simulink model "diagrama_completo"  (R2020b)
settings: Solver=VariableStepAuto  StartTime=0.0  StopTime=25  MaxStep=1e-4  RelTol=1e-4
model workspace (MAT data in the model file):
  Cts = 0.818
  Jeq = 5.65099476805e-06
  Ld = 0.0066
  Lls = 0.0008
  Lq = 0.0058
  Pp = 3
  Rs = 1.02
  Rts_amb = 146.7
  beq = 1.5e-05
  lambda_m = 0.01546
  r = 314.3008
  ws = 15000
  wsv = 30000
values from neighbouring files (symbols this model uses):
  ba = Jeq*n*wpos    (= 0.0113019895361)    [valores.m]
  kotheta = 3*pobs    (= 9600)    [valores.m]
  koTl = (pobs^3)    (= 32768000000)    [valores.m]
  kow = 3*(pobs^2)    (= 30720000)    [valores.m]
  ksa = ba*wpos    (= 9.04159162887)    [valores.m]
  ksia = ksa*wint    (= 2893.30932124)    [valores.m]
  R0 = Lls*pi    (= 4)    [valores.m]
  Rd = Ld*pi    (= 33)    [valores.m]
  Rq = Lq*pi    (= 29)    [valores.m]
undefined symbols (not defined in the file or in its folder): sigbuilder_block
(part 2 of 2)

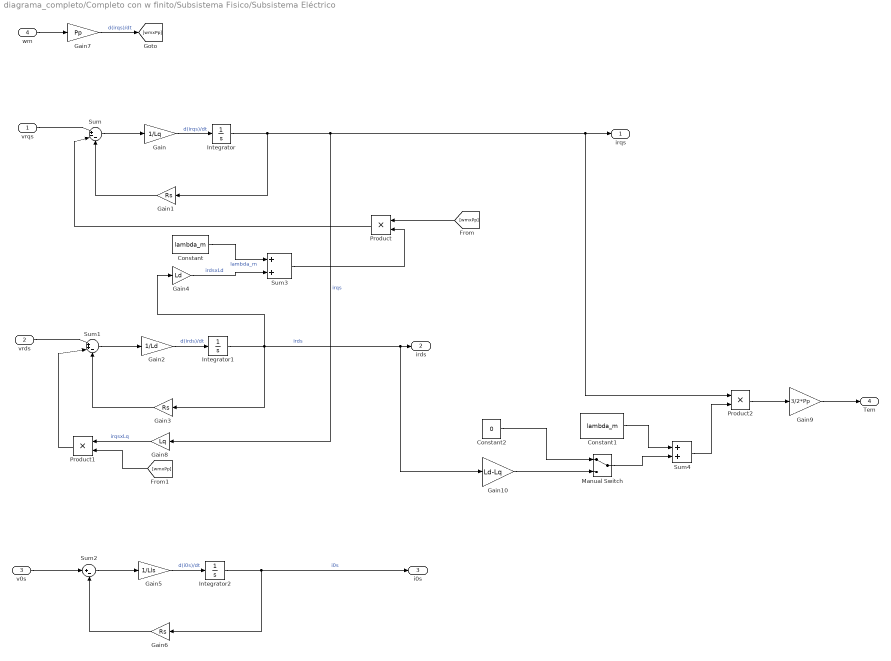
== system diagrama_completo/Completo con w finito/Subsistema Fisico/Subsistema Eléctrico ==
  vrqs : Inport
  vrds : Inport  Port=2
  v0s : Inport  Port=3
  wm : Inport  Port=4
  Constant : Constant  Value=lambda_m
  Constant1 : Constant  Value=lambda_m
  Constant2 : Constant  Value=0
  Gain : Gain  Gain=1/Lq
  Gain1 : Gain  Gain=Rs
  Gain10 : Gain  Gain=Ld-Lq
  Gain2 : Gain  Gain=1/Ld
  Gain3 : Gain  Gain=Rs
  Gain4 : Gain  Gain=Ld
  Gain5 : Gain  Gain=1/Lls
  Gain6 : Gain  Gain=Rs
  Gain7 : Gain  Gain=Pp
  Gain8 : Gain  Gain=Lq
  Gain9 : Gain  Gain=3/2*Pp
  Integrator : Integrator
  Integrator1 : Integrator
  Integrator2 : Integrator
  Manual Switch : ManualSwitch
  Product : Product
  Product1 : Product
  Product2 : Product
  Sum : Sum  Inputs=|+--
  Sum1 : Sum  Inputs=|++-
  Sum2 : Sum  Inputs=|+-
  Sum3 : Sum
  Sum4 : Sum
  irqs : Outport
  irds : Outport  Port=2
  i0s : Outport  Port=3
  Tem : Outport  Port=4
  wires:
  Integrator1/1 -> Gain4/1, Gain3/1, Gain10/1, irds/1  "irds"
  Gain2/1 -> Integrator1/1  "d(irds)/dt"
  Gain3/1 -> Sum1/3
  vrqs/1 -> Sum/1
  vrds/1 -> Sum1/1
  v0s/1 -> Sum2/1
  Gain5/1 -> Integrator2/1  "d(i0s)/dt"
  Integrator2/1 -> Gain6/1, i0s/1  "i0s"
  Gain1/1 -> Sum/3
  Integrator/1 -> Gain1/1, Gain8/1, Product2/1, irqs/1  "irqs"
  Gain/1 -> Integrator/1  "d(irqs)/dt"
  Gain6/1 -> Sum2/2
  Gain4/1 -> Sum3/2  "irdsxLd"
  Constant/1 -> Sum3/1  "lambda_m"
  wm/1 -> Gain7/1
  Gain7/1 -> [wmxPp]  "d(irqs)/dt"
  [wmxPp] -> Product/1
  Product/1 -> Sum/2
  Sum3/1 -> Product/2
  Gain8/1 -> Product1/1  "irqsxLq"
  [wmxPp] -> Product1/2
  Product1/1 -> Sum1/2
  Constant1/1 -> Sum4/1
  Sum4/1 -> Product2/2
  Product2/1 -> Gain9/1
  Gain9/1 -> Tem/1
  Sum/1 -> Gain/1
  Sum1/1 -> Gain2/1
  Sum2/1 -> Gain5/1
  Gain10/1 -> Manual Switch/2
  Constant2/1 -> Manual Switch/1
  Manual Switch/1 -> Sum4/2

== system diagrama_completo/Completo con w finito/Subsistema Fisico/Subsistema Mecánico ==
  Tl : Inport
  Tem : Inport  Port=2
  Gain : Gain  Gain=1/Jeq
  Gain1 : Gain  Gain=beq
  Gain2 : Gain  Gain=1/r
  Integrator : Integrator
  Integrator1 : Integrator
  Sum : Sum  Inputs=-+-
  wm : Outport
  theta_m : Outport  Port=2
  wires:
  Sum/1 -> Gain/1
  Tl/1 -> Gain2/1
  Gain1/1 -> Sum/3
  Integrator/1 -> Gain1/1, wm/1, Integrator1/1  "wm"
  Gain2/1 -> Sum/1
  Gain/1 -> Integrator/1  "acel"
  Integrator1/1 -> theta_m/1  "theta_m"
  Tem/1 -> Sum/2

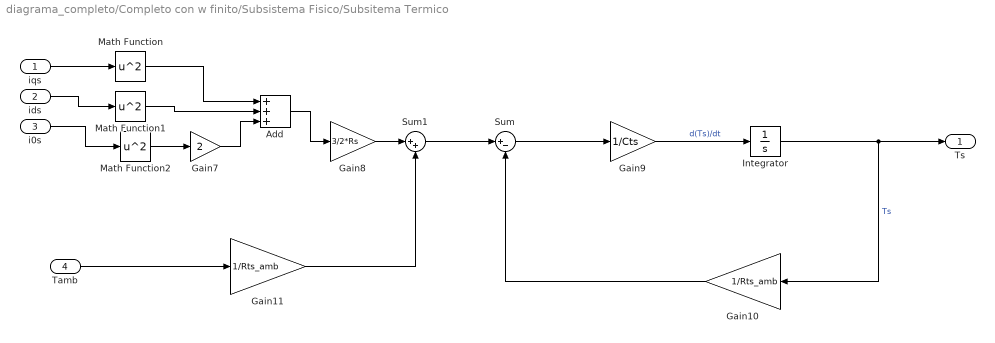
== system diagrama_completo/Completo con w finito/Subsistema Fisico/Subsitema Termico ==
  iqs : Inport
  ids : Inport  Port=2
  i0s : Inport  Port=3
  Tamb : Inport  Port=4
  Add : Sum  Inputs=+++
  Gain10 : Gain  Gain=1/Rts_amb
  Gain11 : Gain  Gain=1/Rts_amb
  Gain7 : Gain  Gain=2
  Gain8 : Gain  Gain=3/2*Rs
  Gain9 : Gain  Gain=1/Cts
  Integrator : Integrator  InitialCondition=40
  Math Function : Math  Operator=square  SaturateOnIntegerOverflow=on
  Math Function1 : Math  Operator=square  SaturateOnIntegerOverflow=on
  Math Function2 : Math  Operator=square  SaturateOnIntegerOverflow=on
  Sum : Sum  Inputs=|+-
  Sum1 : Sum  Inputs=|++
  Ts : Outport
  wires:
  Gain11/1 -> Sum1/2
  Gain8/1 -> Sum1/1
  Add/1 -> Gain8/1
  Gain9/1 -> Integrator/1  "d(Ts)/dt"
  Gain10/1 -> Sum/2
  Integrator/1 -> Gain10/1, Ts/1  "Ts"
  i0s/1 -> Math Function2/1
  Math Function/1 -> Add/1
  ids/1 -> Math Function1/1
  Sum1/1 -> Sum/1
  Gain7/1 -> Add/3
  Sum/1 -> Gain9/1
  Tamb/1 -> Gain11/1
  Math Function2/1 -> Gain7/1
  iqs/1 -> Math Function/1
  Math Function1/1 -> Add/2

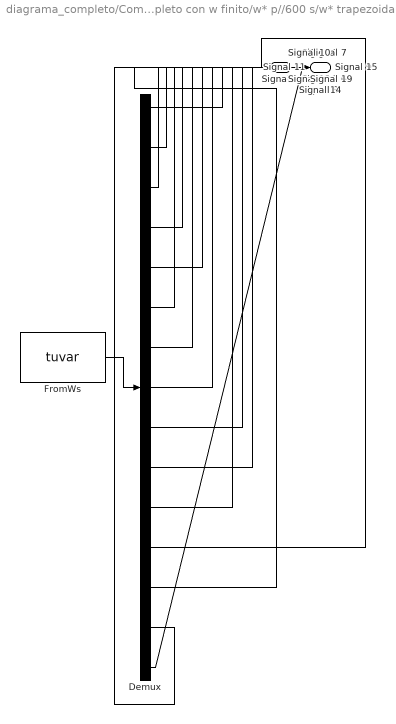
== system diagrama_completo/Completo con w finito/w* p//600 s/w* trapezoidal1 ==
  Demux : Demux  Tag=STV Demux  Outputs=15
      settings: DisplayOption=none
  FromWs : FromWorkspace  Tag=STV FromWs  VariableName=tuvar
      SigBuilderData=|
      | common.afterFinalStr = 'Extrapolate'
      | common.sampleTime = 0
      | dataSet.timeRange = [0 155]
      | dataSet.name = 'Group 1'
      | sbobj.Groups.Name = 'Group 1'
      | sbobj.Groups.Signals(1).Name = 'Signal 1'
      | sbobj.Groups.Signals(1).XData = [0 5 5.2 9.8 10 155]
      | sbobj.Groups.Signals(1).YData = [0 0 1.25663706144 1.25663706144 0 0]
      | sbobj.Groups.Signals(2).Name = 'Signal 2'
      | sbobj.Groups.Signals(2).XData = [0 15 15.2 19.8 20 155]
      | sbobj.Groups.Signals(2).YData = [0 0 -1.25663706144 -1.25663706144 0 0]
      | sbobj.Groups.Signals(3).Name = 'Signal 3'
      | sbobj.Groups.Signals(3).XData = [0 25 25.2 29.8 30 155]
      | sbobj.Groups.Signals(3).YData = [0 0 1.25663706144 1.25663706144 0 0]
      | sbobj.Groups.Signals(4).Name = 'Signal 4'
      | sbobj.Groups.Signals(4).XData = [0 35 35.2 39.8 40 155]
      | sbobj.Groups.Signals(4).YData = [0 0 -1.25663706144 -1.25663706144 0 0]
      | sbobj.Groups.Signals(5).Name = 'Signal 5'
      | sbobj.Groups.Signals(5).XData = [0 45 45.2 49.8 50 155]
      | sbobj.Groups.Signals(5).YData = [0 0 1.25663706144 1.25663706144 0 0]
      | sbobj.Groups.Signals(6).Name = 'Signal 6'
      | sbobj.Groups.Signals(6).XData = [0 55 55.2 59.8 60 155]
      | sbobj.Groups.Signals(6).YData = [0 0 -1.25663706144 -1.25663706144 0 0]
      | sbobj.Groups.Signals(7).Name = 'Signal 7'
      | sbobj.Groups.Signals(7).XData = [0 65 65.2 69.8 70 155]
      | sbobj.Groups.Signals(7).YData = [0 0 1.25663706144 1.25663706144 0 0]
      | sbobj.Groups.Signals(8).Name = 'Signal 8'
      | sbobj.Groups.Signals(8).XData = [0 75 75.2 79.8 80 155]
      | sbobj.Groups.Signals(8).YData = [0 0 -1.25663706144 -1.25663706144 0 0]
      | sbobj.Groups.Signals(9).Name = 'Signal 9'
      | sbobj.Groups.Signals(9).XData = [0 85 85.2 89.8 90 155]
      | sbobj.Groups.Signals(9).YData = [0 0 1.25663706144 1.25663706144 0 0]
      | sbobj.Groups.Signals(10).Name = 'Signal 10'
      | sbobj.Groups.Signals(10).XData = [0 95 95.2 99.8 100 155]
      | sbobj.Groups.Signals(10).YData = [0 0 -1.25663706144 -1.25663706144 0 0]
      | sbobj.Groups.Signals(11).Name = 'Signal 11'
      | sbobj.Groups.Signals(11).XData = [0 105 105.2 109.8 110 155]
      | sbobj.Groups.Signals(11).YData = [0 0 1.25663706144 1.25663706144 0 0]
      | sbobj.Groups.Signals(12).Name = 'Signal 12'
      | sbobj.Groups.Signals(12).XData = [0 115 115.2 119.8 120 155]
      | sbobj.Groups.Signals(12).YData = [0 0 -1.25663706144 -1.25663706144 0 0]
      | sbobj.Groups.Signals(13).Name = 'Signal 14'
      | sbobj.Groups.Signals(13).XData = [0 125 125.2 129.8 130 155]
      | sbobj.Groups.Signals(13).YData = [0 0 1.2566 1.2566 0 0]
      | sbobj.Groups.Signals(14).Name = 'Signal 15'
      | sbobj.Groups.Signals(14).XData = [0 135 135.2 139.8 140 155]
      | sbobj.Groups.Signals(14).YData = [0 0 -1.2566 -1.2566 0 0]
      | sbobj.Groups.Signals(15).Name = 'Signal 19'
      | sbobj.Groups.Signals(15).XData = [0 145 145.2 149.8 150 155]
      | sbobj.Groups.Signals(15).YData = [0 0 1.2566 1.2566 0 0]
      | sbobj.Groups.TimeRange = [0 155]
  Signal 1 : Outport  Tag=STV Outport
  Signal 2 : Outport  Tag=STV Outport  Port=2
  Signal 3 : Outport  Tag=STV Outport  Port=3
  Signal 4 : Outport  Tag=STV Outport  Port=4
  Signal 5 : Outport  Tag=STV Outport  Port=5
  Signal 6 : Outport  Tag=STV Outport  Port=6
  Signal 7 : Outport  Tag=STV Outport  Port=7
  Signal 8 : Outport  Tag=STV Outport  Port=8
  Signal 9 : Outport  Tag=STV Outport  Port=9
  Signal 10 : Outport  Tag=STV Outport  Port=10
  Signal 11 : Outport  Tag=STV Outport  Port=11
  Signal 12 : Outport  Tag=STV Outport  Port=12
  Signal 14 : Outport  Tag=STV Outport  Port=13
  Signal 15 : Outport  Tag=STV Outport  Port=14
  Signal 19 : Outport  Tag=STV Outport  Port=15
  wires:
  FromWs/1 -> Demux/1
  Demux/1 -> Signal 1/1
  Demux/2 -> Signal 2/1
  Demux/3 -> Signal 3/1
  Demux/4 -> Signal 4/1
  Demux/5 -> Signal 5/1
  Demux/6 -> Signal 6/1
  Demux/7 -> Signal 7/1
  Demux/8 -> Signal 8/1
  Demux/9 -> Signal 9/1
  Demux/10 -> Signal 10/1
  Demux/11 -> Signal 11/1
  Demux/12 -> Signal 12/1
  Demux/13 -> Signal 14/1
  Demux/14 -> Signal 15/1
  Demux/15 -> Signal 19/1

== system diagrama_completo/Completo con w finito/w* p//600 s/w* trapezoidal2 ==
  Demux : Demux  Tag=STV Demux  Outputs=15
      settings: DisplayOption=none
  FromWs : FromWorkspace  Tag=STV FromWs  VariableName=tuvar
      SigBuilderData=|
      | common.afterFinalStr = 'Extrapolate'
      | common.sampleTime = 0
      | dataSet.timeRange = [0 305]
      | dataSet.name = 'Group 1'
      | sbobj.Groups.Name = 'Group 1'
      | sbobj.Groups.Signals(1).Name = 'Signal 1'
      | sbobj.Groups.Signals(1).XData = [0 155 155.2 159.8 160 305]
      | sbobj.Groups.Signals(1).YData = [0 0 -1.2566 -1.25663706144 0 0]
      | sbobj.Groups.Signals(2).Name = 'Signal 2'
      | sbobj.Groups.Signals(2).XData = [0 165 165.2 169.8 170 305]
      | sbobj.Groups.Signals(2).YData = [0 0 1.2566 1.2566 0 0]
      | sbobj.Groups.Signals(3).Name = 'Signal 3'
      | sbobj.Groups.Signals(3).XData = [0 175 175.2 179.8 180 305]
      | sbobj.Groups.Signals(3).YData = [0 0 -1.25663706144 -1.2566 0 0]
      | sbobj.Groups.Signals(4).Name = 'Signal 4'
      | sbobj.Groups.Signals(4).XData = [0 185 185.2 189.8 190 305]
      | sbobj.Groups.Signals(4).YData = [0 0 1.2566 1.2566 0 0]
      | sbobj.Groups.Signals(5).Name = 'Signal 5'
      | sbobj.Groups.Signals(5).XData = [0 195 195.2 199.8 200 305]
      | sbobj.Groups.Signals(5).YData = [0 0 -1.2566 -1.2566 0 0]
      | sbobj.Groups.Signals(6).Name = 'Signal 6'
      | sbobj.Groups.Signals(6).XData = [0 205 205.2 209.8 210 305]
      | sbobj.Groups.Signals(6).YData = [0 0 1.2566 1.2566 0 0]
      | sbobj.Groups.Signals(7).Name = 'Signal 7'
      | sbobj.Groups.Signals(7).XData = [0 215 215.2 219.8 220 305]
      | sbobj.Groups.Signals(7).YData = [0 0 -1.2566 -1.2566 0 0]
      | sbobj.Groups.Signals(8).Name = 'Signal 8'
      | sbobj.Groups.Signals(8).XData = [0 225 225.2 229.8 230 305]
      | sbobj.Groups.Signals(8).YData = [0 0 1.2566 1.2566 0 0]
      | sbobj.Groups.Signals(9).Name = 'Signal 9'
      | sbobj.Groups.Signals(9).XData = [0 235 235.2 239.8 240 305]
      | sbobj.Groups.Signals(9).YData = [0 0 -1.2566 -1.2566 0 0]
      | sbobj.Groups.Signals(10).Name = 'Signal 10'
      | sbobj.Groups.Signals(10).XData = [0 245 245.2 249.8 250 305]
      | sbobj.Groups.Signals(10).YData = [0 0 1.25663706144 1.2566 0 0]
      | sbobj.Groups.Signals(11).Name = 'Signal 11'
      | sbobj.Groups.Signals(11).XData = [0 255 255.2 259.8 260 305]
      | sbobj.Groups.Signals(11).YData = [0 0 -1.2566 -1.2566 0 0]
      | sbobj.Groups.Signals(12).Name = 'Signal 12'
      | sbobj.Groups.Signals(12).XData = [0 265 265.2 269.8 270 305]
      | sbobj.Groups.Signals(12).YData = [0 0 1.2566 1.2566 0 0]
      | sbobj.Groups.Signals(13).Name = 'Signal 13'
      | sbobj.Groups.Signals(13).XData = [0 275 275.2 279.8 280 305]
      | sbobj.Groups.Signals(13).YData = [0 0 -1.2566 -1.2566 0 0]
      | sbobj.Groups.Signals(14).Name = 'Signal 14'
      | sbobj.Groups.Signals(14).XData = [0 285 285.2 289.8 290 305]
      | sbobj.Groups.Signals(14).YData = [0 0 1.2566 1.2566 0 0]
      | sbobj.Groups.Signals(15).Name = 'Signal 15'
      | sbobj.Groups.Signals(15).XData = [0 295 295.2 299.8 300 305]
      | sbobj.Groups.Signals(15).YData = [0 0 -1.2566 -1.2566 0 0]
      | sbobj.Groups.TimeRange = [0 305]
  Signal 1 : Outport  Tag=STV Outport
  Signal 2 : Outport  Tag=STV Outport  Port=2
  Signal 3 : Outport  Tag=STV Outport  Port=3
  Signal 4 : Outport  Tag=STV Outport  Port=4
  Signal 5 : Outport  Tag=STV Outport  Port=5
  Signal 6 : Outport  Tag=STV Outport  Port=6
  Signal 7 : Outport  Tag=STV Outport  Port=7
  Signal 8 : Outport  Tag=STV Outport  Port=8
  Signal 9 : Outport  Tag=STV Outport  Port=9
  Signal 10 : Outport  Tag=STV Outport  Port=10
  Signal 11 : Outport  Tag=STV Outport  Port=11
  Signal 12 : Outport  Tag=STV Outport  Port=12
  Signal 13 : Outport  Tag=STV Outport  Port=13
  Signal 14 : Outport  Tag=STV Outport  Port=14
  Signal 15 : Outport  Tag=STV Outport  Port=15
  wires:
  FromWs/1 -> Demux/1
  Demux/1 -> Signal 1/1
  Demux/2 -> Signal 2/1
  Demux/3 -> Signal 3/1
  Demux/4 -> Signal 4/1
  Demux/5 -> Signal 5/1
  Demux/6 -> Signal 6/1
  Demux/7 -> Signal 7/1
  Demux/8 -> Signal 8/1
  Demux/9 -> Signal 9/1
  Demux/10 -> Signal 10/1
  Demux/11 -> Signal 11/1
  Demux/12 -> Signal 12/1
  Demux/13 -> Signal 13/1
  Demux/14 -> Signal 14/1
  Demux/15 -> Signal 15/1

== system diagrama_completo/Completo con w finito/w* p//600 s/w* trapezoidal3 ==
  Demux : Demux  Tag=STV Demux  Outputs=15
      settings: DisplayOption=none
  FromWs : FromWorkspace  Tag=STV FromWs  VariableName=tuvar
      SigBuilderData=|
      | common.afterFinalStr = 'Extrapolate'
      | common.sampleTime = 0
      | dataSet.timeRange = [0 455]
      | dataSet.name = 'Group 1'
      | sbobj.Groups.Name = 'Group 1'
      | sbobj.Groups.Signals(1).Name = 'Signal 1'
      | sbobj.Groups.Signals(1).XData = [0 305 305.2 309.8 310 455]
      | sbobj.Groups.Signals(1).YData = [0 0 1.25663706144 1.25663706144 0 0]
      | sbobj.Groups.Signals(2).Name = 'Signal 2'
      | sbobj.Groups.Signals(2).XData = [0 315 315.2 319.8 320 455]
      | sbobj.Groups.Signals(2).YData = [0 0 -1.25663706144 -1.25663706144 0 0]
      | sbobj.Groups.Signals(3).Name = 'Signal 3'
      | sbobj.Groups.Signals(3).XData = [0 325 325.2 329.8 330 455]
      | sbobj.Groups.Signals(3).YData = [0 0 1.25663706144 1.25663706144 0 0]
      | sbobj.Groups.Signals(4).Name = 'Signal 4'
      | sbobj.Groups.Signals(4).XData = [0 335 335.2 339.8 340 455]
      | sbobj.Groups.Signals(4).YData = [0 0 -1.25663706144 -1.25663706144 0 0]
      | sbobj.Groups.Signals(5).Name = 'Signal 5'
      | sbobj.Groups.Signals(5).XData = [0 345 345.2 349.8 350 455]
      | sbobj.Groups.Signals(5).YData = [0 0 1.25663706144 1.25663706144 0 0]
      | sbobj.Groups.Signals(6).Name = 'Signal 6'
      | sbobj.Groups.Signals(6).XData = [0 355 355.2 359.8 360 455]
      | sbobj.Groups.Signals(6).YData = [0 0 -1.25663706144 -1.25663706144 0 0]
      | sbobj.Groups.Signals(7).Name = 'Signal 7'
      | sbobj.Groups.Signals(7).XData = [0 365 365.2 369.8 370 455]
      | sbobj.Groups.Signals(7).YData = [0 0 1.25663706144 1.25663706144 0 0]
      | sbobj.Groups.Signals(8).Name = 'Signal 8'
      | sbobj.Groups.Signals(8).XData = [0 375 375.2 379.8 380 455]
      | sbobj.Groups.Signals(8).YData = [0 0 -1.25663706144 -1.25663706144 0 0]
      | sbobj.Groups.Signals(9).Name = 'Signal 9'
      | sbobj.Groups.Signals(9).XData = [0 385 385.2 389.8 390 455]
      | sbobj.Groups.Signals(9).YData = [0 0 1.25663706144 1.25663706144 0 0]
      | sbobj.Groups.Signals(10).Name = 'Signal 10'
      | sbobj.Groups.Signals(10).XData = [0 395 395.2 399.8 400 455]
      | sbobj.Groups.Signals(10).YData = [0 0 -1.25663706144 -1.25663706144 0 0]
      | sbobj.Groups.Signals(11).Name = 'Signal 11'
      | sbobj.Groups.Signals(11).XData = [0 405 405.2 409.8 410 455]
      | sbobj.Groups.Signals(11).YData = [0 0 1.25663706144 1.25663706144 0 0]
      | sbobj.Groups.Signals(12).Name = 'Signal 12'
      | sbobj.Groups.Signals(12).XData = [0 415 415.2 419.8 420 455]
      | sbobj.Groups.Signals(12).YData = [0 0 -1.25663706144 -1.25663706144 0 0]
      | sbobj.Groups.Signals(13).Name = 'Signal 13'
      | sbobj.Groups.Signals(13).XData = [0 425 425.2 429.8 430 455]
      | sbobj.Groups.Signals(13).YData = [0 0 1.25663706144 1.25663706144 0 0]
      | sbobj.Groups.Signals(14).Name = 'Signal 14'
      | sbobj.Groups.Signals(14).XData = [0 435 435.2 439.8 440 455]
      | sbobj.Groups.Signals(14).YData = [0 0 -1.25663706144 -1.25663706144 0 0]
      | sbobj.Groups.Signals(15).Name = 'Signal 15'
      | sbobj.Groups.Signals(15).XData = [0 445 445.2 449.8 450 455]
      | sbobj.Groups.Signals(15).YData = [0 0 1.25663706144 1.25663706144 0 0]
      | sbobj.Groups.TimeRange = [0 455]
  Signal 1 : Outport  Tag=STV Outport
  Signal 2 : Outport  Tag=STV Outport  Port=2
  Signal 3 : Outport  Tag=STV Outport  Port=3
  Signal 4 : Outport  Tag=STV Outport  Port=4
  Signal 5 : Outport  Tag=STV Outport  Port=5
  Signal 6 : Outport  Tag=STV Outport  Port=6
  Signal 7 : Outport  Tag=STV Outport  Port=7
  Signal 8 : Outport  Tag=STV Outport  Port=8
  Signal 9 : Outport  Tag=STV Outport  Port=9
  Signal 10 : Outport  Tag=STV Outport  Port=10
  Signal 11 : Outport  Tag=STV Outport  Port=11
  Signal 12 : Outport  Tag=STV Outport  Port=12
  Signal 13 : Outport  Tag=STV Outport  Port=13
  Signal 14 : Outport  Tag=STV Outport  Port=14
  Signal 15 : Outport  Tag=STV Outport  Port=15
  wires:
  FromWs/1 -> Demux/1
  Demux/1 -> Signal 1/1
  Demux/2 -> Signal 2/1
  Demux/3 -> Signal 3/1
  Demux/4 -> Signal 4/1
  Demux/5 -> Signal 5/1
  Demux/6 -> Signal 6/1
  Demux/7 -> Signal 7/1
  Demux/8 -> Signal 8/1
  Demux/9 -> Signal 9/1
  Demux/10 -> Signal 10/1
  Demux/11 -> Signal 11/1
  Demux/12 -> Signal 12/1
  Demux/13 -> Signal 13/1
  Demux/14 -> Signal 14/1
  Demux/15 -> Signal 15/1

== system diagrama_completo/Completo con w finito/w* p//600 s/w* trapezoidal4 ==
  Demux : Demux  Tag=STV Demux  Outputs=15
      settings: DisplayOption=none
  FromWs : FromWorkspace  Tag=STV FromWs  VariableName=tuvar
      SigBuilderData=|
      | common.afterFinalStr = 'Extrapolate'
      | common.sampleTime = 0
      | dataSet.timeRange = [0 605]
      | dataSet.name = 'Group 1'
      | sbobj.Groups.Name = 'Group 1'
      | sbobj.Groups.Signals(1).Name = 'Signal 1'
      | sbobj.Groups.Signals(1).XData = [0 455 455.2 459.8 460 605]
      | sbobj.Groups.Signals(1).YData = [0 0 -1.2566 -1.2566 0 0]
      | sbobj.Groups.Signals(2).Name = 'Signal 2'
      | sbobj.Groups.Signals(2).XData = [0 465 465.2 469.8 470 605]
      | sbobj.Groups.Signals(2).YData = [0 0 1.2566 1.2566 0 0]
      | sbobj.Groups.Signals(3).Name = 'Signal 3'
      | sbobj.Groups.Signals(3).XData = [0 475 475.2 479.8 480 605]
      | sbobj.Groups.Signals(3).YData = [0 0 -1.25663706144 -1.2566 0 0]
      | sbobj.Groups.Signals(4).Name = 'Signal 4'
      | sbobj.Groups.Signals(4).XData = [0 485 485.2 489.8 490 605]
      | sbobj.Groups.Signals(4).YData = [0 0 1.25663706144 1.2566 0 0]
      | sbobj.Groups.Signals(5).Name = 'Signal 5'
      | sbobj.Groups.Signals(5).XData = [0 495 495.2 499.8 500 605]
      | sbobj.Groups.Signals(5).YData = [0 0 -1.2566 -1.2566 0 0]
      | sbobj.Groups.Signals(6).Name = 'Signal 6'
      | sbobj.Groups.Signals(6).XData = [0 505 505.2 509.8 510 605]
      | sbobj.Groups.Signals(6).YData = [0 0 1.2566 1.2566 0 0]
      | sbobj.Groups.Signals(7).Name = 'Signal 7'
      | sbobj.Groups.Signals(7).XData = [0 515 515.2 519.8 520 605]
      | sbobj.Groups.Signals(7).YData = [0 0 -1.25663706144 -1.2566 0 0]
      | sbobj.Groups.Signals(8).Name = 'Signal 8'
      | sbobj.Groups.Signals(8).XData = [0 525 525.2 529.8 530 605]
      | sbobj.Groups.Signals(8).YData = [0 0 1.2566 1.2566 0 0]
      | sbobj.Groups.Signals(9).Name = 'Signal 9'
      | sbobj.Groups.Signals(9).XData = [0 535 535.2 539.8 540 605]
      | sbobj.Groups.Signals(9).YData = [0 0 -1.2566 -1.2566 0 0]
      | sbobj.Groups.Signals(10).Name = 'Signal 10'
      | sbobj.Groups.Signals(10).XData = [0 545 545.2 549.8 550 605]
      | sbobj.Groups.Signals(10).YData = [0 0 1.2566 1.2566 0 0]
      | sbobj.Groups.Signals(11).Name = 'Signal 11'
      | sbobj.Groups.Signals(11).XData = [0 555 555.2 559.8 560 605]
      | sbobj.Groups.Signals(11).YData = [0 0 -1.2566 -1.2566 0 0]
      | sbobj.Groups.Signals(12).Name = 'Signal 12'
      | sbobj.Groups.Signals(12).XData = [0 565 565.2 569.8 570 605]
      | sbobj.Groups.Signals(12).YData = [0 0 1.2566 1.2566 0 0]
      | sbobj.Groups.Signals(13).Name = 'Signal 13'
      | sbobj.Groups.Signals(13).XData = [0 575 575.2 579.8 580 605]
      | sbobj.Groups.Signals(13).YData = [0 0 -1.2566 -1.2566 0 0]
      | sbobj.Groups.Signals(14).Name = 'Signal 14'
      | sbobj.Groups.Signals(14).XData = [0 585 585.2 589.8 590 605]
      | sbobj.Groups.Signals(14).YData = [0 0 1.2566 1.2566 0 0]
      | sbobj.Groups.Signals(15).Name = 'Signal 15'
      | sbobj.Groups.Signals(15).XData = [0 595 595.2 599.8 600 605]
      | sbobj.Groups.Signals(15).YData = [0 0 -1.2566 -1.2566 0 0]
      | sbobj.Groups.TimeRange = [0 605]
  Signal 1 : Outport  Tag=STV Outport
  Signal 2 : Outport  Tag=STV Outport  Port=2
  Signal 3 : Outport  Tag=STV Outport  Port=3
  Signal 4 : Outport  Tag=STV Outport  Port=4
  Signal 5 : Outport  Tag=STV Outport  Port=5
  Signal 6 : Outport  Tag=STV Outport  Port=6
  Signal 7 : Outport  Tag=STV Outport  Port=7
  Signal 8 : Outport  Tag=STV Outport  Port=8
  Signal 9 : Outport  Tag=STV Outport  Port=9
  Signal 10 : Outport  Tag=STV Outport  Port=10
  Signal 11 : Outport  Tag=STV Outport  Port=11
  Signal 12 : Outport  Tag=STV Outport  Port=12
  Signal 13 : Outport  Tag=STV Outport  Port=13
  Signal 14 : Outport  Tag=STV Outport  Port=14
  Signal 15 : Outport  Tag=STV Outport  Port=15
  wires:
  FromWs/1 -> Demux/1
  Demux/1 -> Signal 1/1
  Demux/2 -> Signal 2/1
  Demux/3 -> Signal 3/1
  Demux/4 -> Signal 4/1
  Demux/5 -> Signal 5/1
  Demux/6 -> Signal 6/1
  Demux/7 -> Signal 7/1
  Demux/8 -> Signal 8/1
  Demux/9 -> Signal 9/1
  Demux/10 -> Signal 10/1
  Demux/11 -> Signal 11/1
  Demux/12 -> Signal 12/1
  Demux/13 -> Signal 13/1
  Demux/14 -> Signal 14/1
  Demux/15 -> Signal 15/1

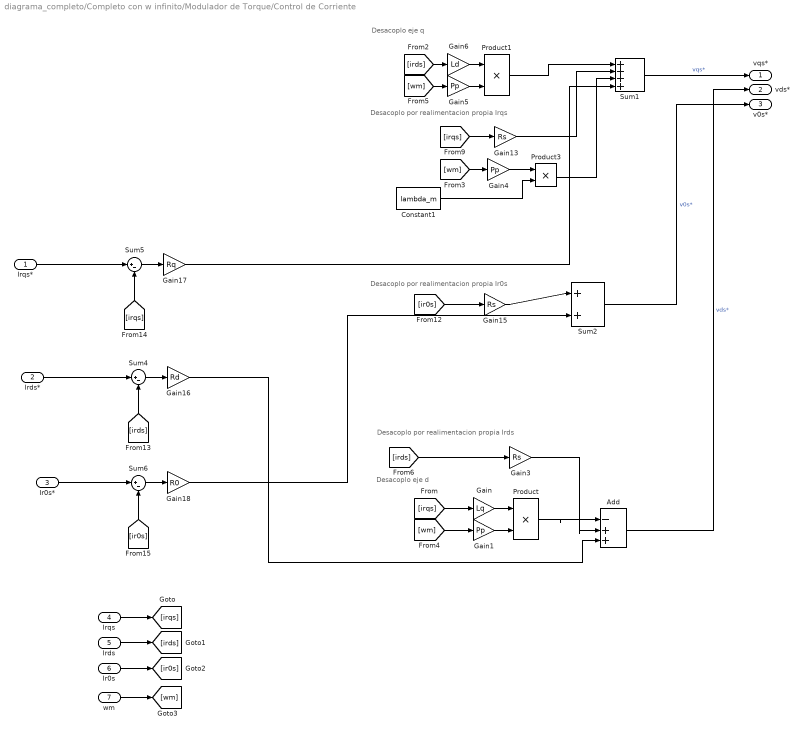
== system diagrama_completo/Completo con w infinito/Modulador de Torque/Control de Corriente ==
  note: Desacoplo por realimentacion propia Ir0s
  note: Desacoplo por realimentacion propia Irqs
  note: Desacoplo por realimentacion propia Irds
  note: Desacoplo eje d
  note: Desacoplo eje q
  Irqs* : Inport
  Irds* : Inport  Port=2
  Ir0s* : Inport  Port=3
  Irqs : Inport  Port=4
  Irds : Inport  Port=5
  Ir0s : Inport  Port=6
  wm : Inport  Port=7
  Add : Sum  Inputs=|-++
  Constant1 : Constant  Value=lambda_m
  Gain : Gain  Gain=Lq
  Gain1 : Gain  Gain=Pp
  Gain13 : Gain  Gain=Rs
  Gain15 : Gain  Gain=Rs
  Gain16 : Gain  Gain=Rd
  Gain17 : Gain  Gain=Rq
  Gain18 : Gain  Gain=R0
  Gain3 : Gain  Gain=Rs
  Gain4 : Gain  Gain=Pp
  Gain5 : Gain  Gain=Pp
  Gain6 : Gain  Gain=Ld
  Product : Product
  Product1 : Product
  Product3 : Product
  Sum1 : Sum  Inputs=|++++
  Sum2 : Sum  Inputs=|++
  Sum4 : Sum  Inputs=|+-
  Sum5 : Sum  Inputs=|+-
  Sum6 : Sum  Inputs=|+-
  vqs* : Outport
  vds* : Outport  Port=2
  v0s* : Outport  Port=3
  wires:
  [ir0s] -> Sum6/2
  Sum2/1 -> v0s*/1  "v0s*"
  Irqs*/1 -> Sum5/1
  Ir0s*/1 -> Sum6/1
  Gain3/1 -> Add/2
  [irqs] -> Gain13/1
  [irds] -> Sum4/2
  [ir0s] -> Gain15/1
  Sum5/1 -> Gain17/1
  [irqs] -> Sum5/2
  [irds] -> Gain3/1
  Gain13/1 -> Sum1/2
  Sum6/1 -> Gain18/1
  Irds*/1 -> Sum4/1
  Gain15/1 -> Sum2/1
  Gain18/1 -> Sum2/2
  Gain17/1 -> Sum1/4
  Product1/1 -> Sum1/1
  Product/1 -> Add/1
  Gain5/1 -> Product1/2
  Gain/1 -> Product/1
  Gain4/1 -> Product3/1
  Sum4/1 -> Gain16/1
  Constant1/1 -> Product3/2
  Product3/1 -> Sum1/3
  Add/1 -> vds*/1  "vds*"
  Sum1/1 -> vqs*/1  "vqs*"
  Irqs/1 -> [irqs]
  Irds/1 -> [irds]
  Ir0s/1 -> [ir0s]
  [irqs] -> Gain/1
  Gain1/1 -> Product/2
  [wm] -> Gain1/1
  wm/1 -> [wm]
  [wm] -> Gain4/1
  [wm] -> Gain5/1
  [irds] -> Gain6/1
  Gain6/1 -> Product1/1
  Gain16/1 -> Add/3

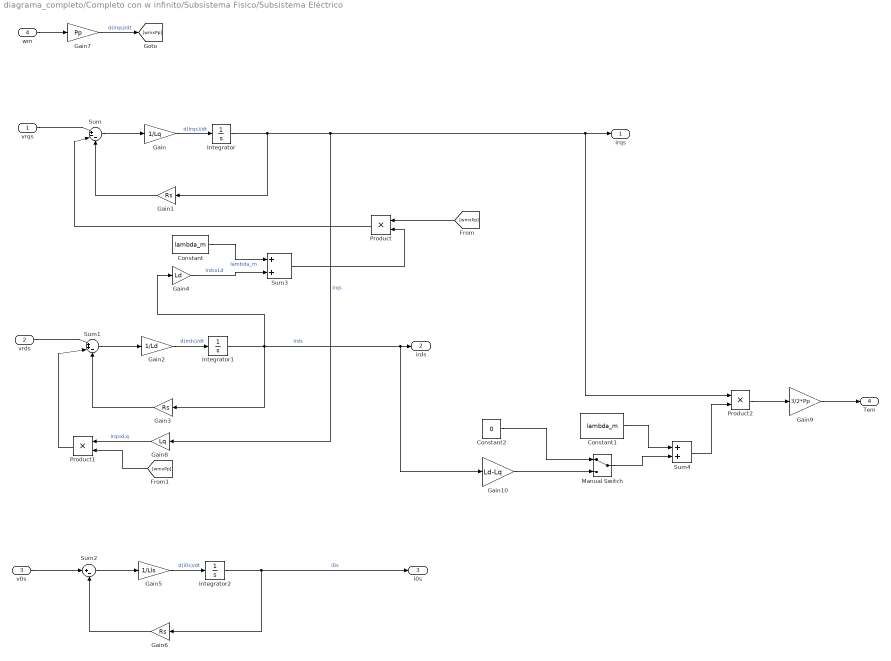
== system diagrama_completo/Completo con w infinito/Subsistema Fisico/Subsistema Eléctrico ==
  vrqs : Inport
  vrds : Inport  Port=2
  v0s : Inport  Port=3
  wm : Inport  Port=4
  Constant : Constant  Value=lambda_m
  Constant1 : Constant  Value=lambda_m
  Constant2 : Constant  Value=0
  Gain : Gain  Gain=1/Lq
  Gain1 : Gain  Gain=Rs
  Gain10 : Gain  Gain=Ld-Lq
  Gain2 : Gain  Gain=1/Ld
  Gain3 : Gain  Gain=Rs
  Gain4 : Gain  Gain=Ld
  Gain5 : Gain  Gain=1/Lls
  Gain6 : Gain  Gain=Rs
  Gain7 : Gain  Gain=Pp
  Gain8 : Gain  Gain=Lq
  Gain9 : Gain  Gain=3/2*Pp
  Integrator : Integrator
  Integrator1 : Integrator
  Integrator2 : Integrator
  Manual Switch : ManualSwitch
  Product : Product
  Product1 : Product
  Product2 : Product
  Sum : Sum  Inputs=|+--
  Sum1 : Sum  Inputs=|++-
  Sum2 : Sum  Inputs=|+-
  Sum3 : Sum
  Sum4 : Sum
  irqs : Outport
  irds : Outport  Port=2
  i0s : Outport  Port=3
  Tem : Outport  Port=4
  wires:
  Integrator1/1 -> Gain4/1, Gain3/1, Gain10/1, irds/1  "irds"
  Gain2/1 -> Integrator1/1  "d(irds)/dt"
  Gain3/1 -> Sum1/3
  vrqs/1 -> Sum/1
  vrds/1 -> Sum1/1
  v0s/1 -> Sum2/1
  Gain5/1 -> Integrator2/1  "d(i0s)/dt"
  Integrator2/1 -> Gain6/1, i0s/1  "i0s"
  Gain1/1 -> Sum/3
  Integrator/1 -> Gain1/1, Gain8/1, Product2/1, irqs/1  "irqs"
  Gain/1 -> Integrator/1  "d(irqs)/dt"
  Gain6/1 -> Sum2/2
  Gain4/1 -> Sum3/2  "irdsxLd"
  Constant/1 -> Sum3/1  "lambda_m"
  wm/1 -> Gain7/1
  Gain7/1 -> [wmxPp]  "d(irqs)/dt"
  [wmxPp] -> Product/1
  Product/1 -> Sum/2
  Sum3/1 -> Product/2
  Gain8/1 -> Product1/1  "irqsxLq"
  [wmxPp] -> Product1/2
  Product1/1 -> Sum1/2
  Constant1/1 -> Sum4/1
  Sum4/1 -> Product2/2
  Product2/1 -> Gain9/1
  Gain9/1 -> Tem/1
  Sum/1 -> Gain/1
  Sum1/1 -> Gain2/1
  Sum2/1 -> Gain5/1
  Gain10/1 -> Manual Switch/2
  Constant2/1 -> Manual Switch/1
  Manual Switch/1 -> Sum4/2

== system diagrama_completo/Completo con w infinito/Subsistema Fisico/Subsistema Mecánico ==
  Tl : Inport
  Tem : Inport  Port=2
  Gain : Gain  Gain=1/Jeq
  Gain1 : Gain  Gain=beq
  Gain2 : Gain  Gain=1/r
  Integrator : Integrator
  Integrator1 : Integrator
  Sum : Sum  Inputs=-+-
  wm : Outport
  theta_m : Outport  Port=2
  wires:
  Sum/1 -> Gain/1
  Tl/1 -> Gain2/1
  Gain1/1 -> Sum/3
  Integrator/1 -> Gain1/1, wm/1, Integrator1/1  "wm"
  Gain2/1 -> Sum/1
  Gain/1 -> Integrator/1  "acel"
  Integrator1/1 -> theta_m/1  "theta_m"
  Tem/1 -> Sum/2

== system diagrama_completo/Completo con w infinito/Subsistema Fisico/Subsitema Termico ==
  iqs : Inport
  ids : Inport  Port=2
  i0s : Inport  Port=3
  Tamb : Inport  Port=4
  Add : Sum  Inputs=+++
  Gain10 : Gain  Gain=1/Rts_amb
  Gain11 : Gain  Gain=1/Rts_amb
  Gain7 : Gain  Gain=2
  Gain8 : Gain  Gain=3/2*Rs
  Gain9 : Gain  Gain=1/Cts
  Integrator : Integrator  InitialCondition=40
  Math Function : Math  Operator=square  SaturateOnIntegerOverflow=on
  Math Function1 : Math  Operator=square  SaturateOnIntegerOverflow=on
  Math Function2 : Math  Operator=square  SaturateOnIntegerOverflow=on
  Sum : Sum  Inputs=|+-
  Sum1 : Sum  Inputs=|++
  Ts : Outport
  wires:
  Gain11/1 -> Sum1/2
  Gain8/1 -> Sum1/1
  Add/1 -> Gain8/1
  Gain9/1 -> Integrator/1  "d(Ts)/dt"
  Gain10/1 -> Sum/2
  Integrator/1 -> Gain10/1, Ts/1  "Ts"
  i0s/1 -> Math Function2/1
  Math Function/1 -> Add/1
  ids/1 -> Math Function1/1
  Sum1/1 -> Sum/1
  Gain7/1 -> Add/3
  Sum/1 -> Gain9/1
  Tamb/1 -> Gain11/1
  Math Function2/1 -> Gain7/1
  iqs/1 -> Math Function/1
  Math Function1/1 -> Add/2

== system diagrama_completo/Completo con w infinito/w* p//600 s/w* trapezoidal1 ==
  Demux : Demux  Tag=STV Demux  Outputs=15
      settings: DisplayOption=none
  FromWs : FromWorkspace  Tag=STV FromWs  VariableName=tuvar
      SigBuilderData=|
      | common.afterFinalStr = 'Extrapolate'
      | common.sampleTime = 0
      | dataSet.timeRange = [0 155]
      | dataSet.name = 'Group 1'
      | sbobj.Groups.Name = 'Group 1'
      | sbobj.Groups.Signals(1).Name = 'Signal 1'
      | sbobj.Groups.Signals(1).XData = [0 5 5.2 9.8 10 155]
      | sbobj.Groups.Signals(1).YData = [0 0 1.25663706144 1.25663706144 0 0]
      | sbobj.Groups.Signals(2).Name = 'Signal 2'
      | sbobj.Groups.Signals(2).XData = [0 15 15.2 19.8 20 155]
      | sbobj.Groups.Signals(2).YData = [0 0 -1.25663706144 -1.25663706144 0 0]
      | sbobj.Groups.Signals(3).Name = 'Signal 3'
      | sbobj.Groups.Signals(3).XData = [0 25 25.2 29.8 30 155]
      | sbobj.Groups.Signals(3).YData = [0 0 1.25663706144 1.25663706144 0 0]
      | sbobj.Groups.Signals(4).Name = 'Signal 4'
      | sbobj.Groups.Signals(4).XData = [0 35 35.2 39.8 40 155]
      | sbobj.Groups.Signals(4).YData = [0 0 -1.25663706144 -1.25663706144 0 0]
      | sbobj.Groups.Signals(5).Name = 'Signal 5'
      | sbobj.Groups.Signals(5).XData = [0 45 45.2 49.8 50 155]
      | sbobj.Groups.Signals(5).YData = [0 0 1.25663706144 1.25663706144 0 0]
      | sbobj.Groups.Signals(6).Name = 'Signal 6'
      | sbobj.Groups.Signals(6).XData = [0 55 55.2 59.8 60 155]
      | sbobj.Groups.Signals(6).YData = [0 0 -1.25663706144 -1.25663706144 0 0]
      | sbobj.Groups.Signals(7).Name = 'Signal 7'
      | sbobj.Groups.Signals(7).XData = [0 65 65.2 69.8 70 155]
      | sbobj.Groups.Signals(7).YData = [0 0 1.25663706144 1.25663706144 0 0]
      | sbobj.Groups.Signals(8).Name = 'Signal 8'
      | sbobj.Groups.Signals(8).XData = [0 75 75.2 79.8 80 155]
      | sbobj.Groups.Signals(8).YData = [0 0 -1.25663706144 -1.25663706144 0 0]
      | sbobj.Groups.Signals(9).Name = 'Signal 9'
      | sbobj.Groups.Signals(9).XData = [0 85 85.2 89.8 90 155]
      | sbobj.Groups.Signals(9).YData = [0 0 1.25663706144 1.25663706144 0 0]
      | sbobj.Groups.Signals(10).Name = 'Signal 10'
      | sbobj.Groups.Signals(10).XData = [0 95 95.2 99.8 100 155]
      | sbobj.Groups.Signals(10).YData = [0 0 -1.25663706144 -1.25663706144 0 0]
      | sbobj.Groups.Signals(11).Name = 'Signal 11'
      | sbobj.Groups.Signals(11).XData = [0 105 105.2 109.8 110 155]
      | sbobj.Groups.Signals(11).YData = [0 0 1.25663706144 1.25663706144 0 0]
      | sbobj.Groups.Signals(12).Name = 'Signal 12'
      | sbobj.Groups.Signals(12).XData = [0 115 115.2 119.8 120 155]
      | sbobj.Groups.Signals(12).YData = [0 0 -1.25663706144 -1.25663706144 0 0]
      | sbobj.Groups.Signals(13).Name = 'Signal 14'
      | sbobj.Groups.Signals(13).XData = [0 125 125.2 129.8 130 155]
      | sbobj.Groups.Signals(13).YData = [0 0 1.2566 1.2566 0 0]
      | sbobj.Groups.Signals(14).Name = 'Signal 15'
      | sbobj.Groups.Signals(14).XData = [0 135 135.2 139.8 140 155]
      | sbobj.Groups.Signals(14).YData = [0 0 -1.2566 -1.2566 0 0]
      | sbobj.Groups.Signals(15).Name = 'Signal 19'
      | sbobj.Groups.Signals(15).XData = [0 145 145.2 149.8 150 155]
      | sbobj.Groups.Signals(15).YData = [0 0 1.2566 1.2566 0 0]
      | sbobj.Groups.TimeRange = [0 155]
  Signal 1 : Outport  Tag=STV Outport
  Signal 2 : Outport  Tag=STV Outport  Port=2
  Signal 3 : Outport  Tag=STV Outport  Port=3
  Signal 4 : Outport  Tag=STV Outport  Port=4
  Signal 5 : Outport  Tag=STV Outport  Port=5
  Signal 6 : Outport  Tag=STV Outport  Port=6
  Signal 7 : Outport  Tag=STV Outport  Port=7
  Signal 8 : Outport  Tag=STV Outport  Port=8
  Signal 9 : Outport  Tag=STV Outport  Port=9
  Signal 10 : Outport  Tag=STV Outport  Port=10
  Signal 11 : Outport  Tag=STV Outport  Port=11
  Signal 12 : Outport  Tag=STV Outport  Port=12
  Signal 14 : Outport  Tag=STV Outport  Port=13
  Signal 15 : Outport  Tag=STV Outport  Port=14
  Signal 19 : Outport  Tag=STV Outport  Port=15
  wires:
  FromWs/1 -> Demux/1
  Demux/1 -> Signal 1/1
  Demux/2 -> Signal 2/1
  Demux/3 -> Signal 3/1
  Demux/4 -> Signal 4/1
  Demux/5 -> Signal 5/1
  Demux/6 -> Signal 6/1
  Demux/7 -> Signal 7/1
  Demux/8 -> Signal 8/1
  Demux/9 -> Signal 9/1
  Demux/10 -> Signal 10/1
  Demux/11 -> Signal 11/1
  Demux/12 -> Signal 12/1
  Demux/13 -> Signal 14/1
  Demux/14 -> Signal 15/1
  Demux/15 -> Signal 19/1

== system diagrama_completo/Completo con w infinito/w* p//600 s/w* trapezoidal2 ==
  Demux : Demux  Tag=STV Demux  Outputs=15
      settings: DisplayOption=none
  FromWs : FromWorkspace  Tag=STV FromWs  VariableName=tuvar
      SigBuilderData=|
      | common.afterFinalStr = 'Extrapolate'
      | common.sampleTime = 0
      | dataSet.timeRange = [0 305]
      | dataSet.name = 'Group 1'
      | sbobj.Groups.Name = 'Group 1'
      | sbobj.Groups.Signals(1).Name = 'Signal 1'
      | sbobj.Groups.Signals(1).XData = [0 155 155.2 159.8 160 305]
      | sbobj.Groups.Signals(1).YData = [0 0 -1.2566 -1.25663706144 0 0]
      | sbobj.Groups.Signals(2).Name = 'Signal 2'
      | sbobj.Groups.Signals(2).XData = [0 165 165.2 169.8 170 305]
      | sbobj.Groups.Signals(2).YData = [0 0 1.2566 1.2566 0 0]
      | sbobj.Groups.Signals(3).Name = 'Signal 3'
      | sbobj.Groups.Signals(3).XData = [0 175 175.2 179.8 180 305]
      | sbobj.Groups.Signals(3).YData = [0 0 -1.25663706144 -1.2566 0 0]
      | sbobj.Groups.Signals(4).Name = 'Signal 4'
      | sbobj.Groups.Signals(4).XData = [0 185 185.2 189.8 190 305]
      | sbobj.Groups.Signals(4).YData = [0 0 1.2566 1.2566 0 0]
      | sbobj.Groups.Signals(5).Name = 'Signal 5'
      | sbobj.Groups.Signals(5).XData = [0 195 195.2 199.8 200 305]
      | sbobj.Groups.Signals(5).YData = [0 0 -1.2566 -1.2566 0 0]
      | sbobj.Groups.Signals(6).Name = 'Signal 6'
      | sbobj.Groups.Signals(6).XData = [0 205 205.2 209.8 210 305]
      | sbobj.Groups.Signals(6).YData = [0 0 1.2566 1.2566 0 0]
      | sbobj.Groups.Signals(7).Name = 'Signal 7'
      | sbobj.Groups.Signals(7).XData = [0 215 215.2 219.8 220 305]
      | sbobj.Groups.Signals(7).YData = [0 0 -1.2566 -1.2566 0 0]
      | sbobj.Groups.Signals(8).Name = 'Signal 8'
      | sbobj.Groups.Signals(8).XData = [0 225 225.2 229.8 230 305]
      | sbobj.Groups.Signals(8).YData = [0 0 1.2566 1.2566 0 0]
      | sbobj.Groups.Signals(9).Name = 'Signal 9'
      | sbobj.Groups.Signals(9).XData = [0 235 235.2 239.8 240 305]
      | sbobj.Groups.Signals(9).YData = [0 0 -1.2566 -1.2566 0 0]
      | sbobj.Groups.Signals(10).Name = 'Signal 10'
      | sbobj.Groups.Signals(10).XData = [0 245 245.2 249.8 250 305]
      | sbobj.Groups.Signals(10).YData = [0 0 1.25663706144 1.2566 0 0]
      | sbobj.Groups.Signals(11).Name = 'Signal 11'
      | sbobj.Groups.Signals(11).XData = [0 255 255.2 259.8 260 305]
      | sbobj.Groups.Signals(11).YData = [0 0 -1.2566 -1.2566 0 0]
      | sbobj.Groups.Signals(12).Name = 'Signal 12'
      | sbobj.Groups.Signals(12).XData = [0 265 265.2 269.8 270 305]
      | sbobj.Groups.Signals(12).YData = [0 0 1.2566 1.2566 0 0]
      | sbobj.Groups.Signals(13).Name = 'Signal 13'
      | sbobj.Groups.Signals(13).XData = [0 275 275.2 279.8 280 305]
      | sbobj.Groups.Signals(13).YData = [0 0 -1.2566 -1.2566 0 0]
      | sbobj.Groups.Signals(14).Name = 'Signal 14'
      | sbobj.Groups.Signals(14).XData = [0 285 285.2 289.8 290 305]
      | sbobj.Groups.Signals(14).YData = [0 0 1.2566 1.2566 0 0]
      | sbobj.Groups.Signals(15).Name = 'Signal 15'
      | sbobj.Groups.Signals(15).XData = [0 295 295.2 299.8 300 305]
      | sbobj.Groups.Signals(15).YData = [0 0 -1.2566 -1.2566 0 0]
      | sbobj.Groups.TimeRange = [0 305]
  Signal 1 : Outport  Tag=STV Outport
  Signal 2 : Outport  Tag=STV Outport  Port=2
  Signal 3 : Outport  Tag=STV Outport  Port=3
  Signal 4 : Outport  Tag=STV Outport  Port=4
  Signal 5 : Outport  Tag=STV Outport  Port=5
  Signal 6 : Outport  Tag=STV Outport  Port=6
  Signal 7 : Outport  Tag=STV Outport  Port=7
  Signal 8 : Outport  Tag=STV Outport  Port=8
  Signal 9 : Outport  Tag=STV Outport  Port=9
  Signal 10 : Outport  Tag=STV Outport  Port=10
  Signal 11 : Outport  Tag=STV Outport  Port=11
  Signal 12 : Outport  Tag=STV Outport  Port=12
  Signal 13 : Outport  Tag=STV Outport  Port=13
  Signal 14 : Outport  Tag=STV Outport  Port=14
  Signal 15 : Outport  Tag=STV Outport  Port=15
  wires:
  FromWs/1 -> Demux/1
  Demux/1 -> Signal 1/1
  Demux/2 -> Signal 2/1
  Demux/3 -> Signal 3/1
  Demux/4 -> Signal 4/1
  Demux/5 -> Signal 5/1
  Demux/6 -> Signal 6/1
  Demux/7 -> Signal 7/1
  Demux/8 -> Signal 8/1
  Demux/9 -> Signal 9/1
  Demux/10 -> Signal 10/1
  Demux/11 -> Signal 11/1
  Demux/12 -> Signal 12/1
  Demux/13 -> Signal 13/1
  Demux/14 -> Signal 14/1
  Demux/15 -> Signal 15/1

== system diagrama_completo/Completo con w infinito/w* p//600 s/w* trapezoidal3 ==
  Demux : Demux  Tag=STV Demux  Outputs=15
      settings: DisplayOption=none
  FromWs : FromWorkspace  Tag=STV FromWs  VariableName=tuvar
      SigBuilderData=|
      | common.afterFinalStr = 'Extrapolate'
      | common.sampleTime = 0
      | dataSet.timeRange = [0 455]
      | dataSet.name = 'Group 1'
      | sbobj.Groups.Name = 'Group 1'
      | sbobj.Groups.Signals(1).Name = 'Signal 1'
      | sbobj.Groups.Signals(1).XData = [0 305 305.2 309.8 310 455]
      | sbobj.Groups.Signals(1).YData = [0 0 1.25663706144 1.25663706144 0 0]
      | sbobj.Groups.Signals(2).Name = 'Signal 2'
      | sbobj.Groups.Signals(2).XData = [0 315 315.2 319.8 320 455]
      | sbobj.Groups.Signals(2).YData = [0 0 -1.25663706144 -1.25663706144 0 0]
      | sbobj.Groups.Signals(3).Name = 'Signal 3'
      | sbobj.Groups.Signals(3).XData = [0 325 325.2 329.8 330 455]
      | sbobj.Groups.Signals(3).YData = [0 0 1.25663706144 1.25663706144 0 0]
      | sbobj.Groups.Signals(4).Name = 'Signal 4'
      | sbobj.Groups.Signals(4).XData = [0 335 335.2 339.8 340 455]
      | sbobj.Groups.Signals(4).YData = [0 0 -1.25663706144 -1.25663706144 0 0]
      | sbobj.Groups.Signals(5).Name = 'Signal 5'
      | sbobj.Groups.Signals(5).XData = [0 345 345.2 349.8 350 455]
      | sbobj.Groups.Signals(5).YData = [0 0 1.25663706144 1.25663706144 0 0]
      | sbobj.Groups.Signals(6).Name = 'Signal 6'
      | sbobj.Groups.Signals(6).XData = [0 355 355.2 359.8 360 455]
      | sbobj.Groups.Signals(6).YData = [0 0 -1.25663706144 -1.25663706144 0 0]
      | sbobj.Groups.Signals(7).Name = 'Signal 7'
      | sbobj.Groups.Signals(7).XData = [0 365 365.2 369.8 370 455]
      | sbobj.Groups.Signals(7).YData = [0 0 1.25663706144 1.25663706144 0 0]
      | sbobj.Groups.Signals(8).Name = 'Signal 8'
      | sbobj.Groups.Signals(8).XData = [0 375 375.2 379.8 380 455]
      | sbobj.Groups.Signals(8).YData = [0 0 -1.25663706144 -1.25663706144 0 0]
      | sbobj.Groups.Signals(9).Name = 'Signal 9'
      | sbobj.Groups.Signals(9).XData = [0 385 385.2 389.8 390 455]
      | sbobj.Groups.Signals(9).YData = [0 0 1.25663706144 1.25663706144 0 0]
      | sbobj.Groups.Signals(10).Name = 'Signal 10'
      | sbobj.Groups.Signals(10).XData = [0 395 395.2 399.8 400 455]
      | sbobj.Groups.Signals(10).YData = [0 0 -1.25663706144 -1.25663706144 0 0]
      | sbobj.Groups.Signals(11).Name = 'Signal 11'
      | sbobj.Groups.Signals(11).XData = [0 405 405.2 409.8 410 455]
      | sbobj.Groups.Signals(11).YData = [0 0 1.25663706144 1.25663706144 0 0]
      | sbobj.Groups.Signals(12).Name = 'Signal 12'
      | sbobj.Groups.Signals(12).XData = [0 415 415.2 419.8 420 455]
      | sbobj.Groups.Signals(12).YData = [0 0 -1.25663706144 -1.25663706144 0 0]
      | sbobj.Groups.Signals(13).Name = 'Signal 13'
      | sbobj.Groups.Signals(13).XData = [0 425 425.2 429.8 430 455]
      | sbobj.Groups.Signals(13).YData = [0 0 1.25663706144 1.25663706144 0 0]
      | sbobj.Groups.Signals(14).Name = 'Signal 14'
      | sbobj.Groups.Signals(14).XData = [0 435 435.2 439.8 440 455]
      | sbobj.Groups.Signals(14).YData = [0 0 -1.25663706144 -1.25663706144 0 0]
      | sbobj.Groups.Signals(15).Name = 'Signal 15'
      | sbobj.Groups.Signals(15).XData = [0 445 445.2 449.8 450 455]
      | sbobj.Groups.Signals(15).YData = [0 0 1.25663706144 1.25663706144 0 0]
      | sbobj.Groups.TimeRange = [0 455]
  Signal 1 : Outport  Tag=STV Outport
  Signal 2 : Outport  Tag=STV Outport  Port=2
  Signal 3 : Outport  Tag=STV Outport  Port=3
  Signal 4 : Outport  Tag=STV Outport  Port=4
  Signal 5 : Outport  Tag=STV Outport  Port=5
  Signal 6 : Outport  Tag=STV Outport  Port=6
  Signal 7 : Outport  Tag=STV Outport  Port=7
  Signal 8 : Outport  Tag=STV Outport  Port=8
  Signal 9 : Outport  Tag=STV Outport  Port=9
  Signal 10 : Outport  Tag=STV Outport  Port=10
  Signal 11 : Outport  Tag=STV Outport  Port=11
  Signal 12 : Outport  Tag=STV Outport  Port=12
  Signal 13 : Outport  Tag=STV Outport  Port=13
  Signal 14 : Outport  Tag=STV Outport  Port=14
  Signal 15 : Outport  Tag=STV Outport  Port=15
  wires:
  FromWs/1 -> Demux/1
  Demux/1 -> Signal 1/1
  Demux/2 -> Signal 2/1
  Demux/3 -> Signal 3/1
  Demux/4 -> Signal 4/1
  Demux/5 -> Signal 5/1
  Demux/6 -> Signal 6/1
  Demux/7 -> Signal 7/1
  Demux/8 -> Signal 8/1
  Demux/9 -> Signal 9/1
  Demux/10 -> Signal 10/1
  Demux/11 -> Signal 11/1
  Demux/12 -> Signal 12/1
  Demux/13 -> Signal 13/1
  Demux/14 -> Signal 14/1
  Demux/15 -> Signal 15/1

== system diagrama_completo/Completo con w infinito/w* p//600 s/w* trapezoidal4 ==
  Demux : Demux  Tag=STV Demux  Outputs=15
      settings: DisplayOption=none
  FromWs : FromWorkspace  Tag=STV FromWs  VariableName=tuvar
      SigBuilderData=|
      | common.afterFinalStr = 'Extrapolate'
      | common.sampleTime = 0
      | dataSet.timeRange = [0 605]
      | dataSet.name = 'Group 1'
      | sbobj.Groups.Name = 'Group 1'
      | sbobj.Groups.Signals(1).Name = 'Signal 1'
      | sbobj.Groups.Signals(1).XData = [0 455 455.2 459.8 460 605]
      | sbobj.Groups.Signals(1).YData = [0 0 -1.2566 -1.2566 0 0]
      | sbobj.Groups.Signals(2).Name = 'Signal 2'
      | sbobj.Groups.Signals(2).XData = [0 465 465.2 469.8 470 605]
      | sbobj.Groups.Signals(2).YData = [0 0 1.2566 1.2566 0 0]
      | sbobj.Groups.Signals(3).Name = 'Signal 3'
      | sbobj.Groups.Signals(3).XData = [0 475 475.2 479.8 480 605]
      | sbobj.Groups.Signals(3).YData = [0 0 -1.25663706144 -1.2566 0 0]
      | sbobj.Groups.Signals(4).Name = 'Signal 4'
      | sbobj.Groups.Signals(4).XData = [0 485 485.2 489.8 490 605]
      | sbobj.Groups.Signals(4).YData = [0 0 1.25663706144 1.2566 0 0]
      | sbobj.Groups.Signals(5).Name = 'Signal 5'
      | sbobj.Groups.Signals(5).XData = [0 495 495.2 499.8 500 605]
      | sbobj.Groups.Signals(5).YData = [0 0 -1.2566 -1.2566 0 0]
      | sbobj.Groups.Signals(6).Name = 'Signal 6'
      | sbobj.Groups.Signals(6).XData = [0 505 505.2 509.8 510 605]
      | sbobj.Groups.Signals(6).YData = [0 0 1.2566 1.2566 0 0]
      | sbobj.Groups.Signals(7).Name = 'Signal 7'
      | sbobj.Groups.Signals(7).XData = [0 515 515.2 519.8 520 605]
      | sbobj.Groups.Signals(7).YData = [0 0 -1.25663706144 -1.2566 0 0]
      | sbobj.Groups.Signals(8).Name = 'Signal 8'
      | sbobj.Groups.Signals(8).XData = [0 525 525.2 529.8 530 605]
      | sbobj.Groups.Signals(8).YData = [0 0 1.2566 1.2566 0 0]
      | sbobj.Groups.Signals(9).Name = 'Signal 9'
      | sbobj.Groups.Signals(9).XData = [0 535 535.2 539.8 540 605]
      | sbobj.Groups.Signals(9).YData = [0 0 -1.2566 -1.2566 0 0]
      | sbobj.Groups.Signals(10).Name = 'Signal 10'
      | sbobj.Groups.Signals(10).XData = [0 545 545.2 549.8 550 605]
      | sbobj.Groups.Signals(10).YData = [0 0 1.2566 1.2566 0 0]
      | sbobj.Groups.Signals(11).Name = 'Signal 11'
      | sbobj.Groups.Signals(11).XData = [0 555 555.2 559.8 560 605]
      | sbobj.Groups.Signals(11).YData = [0 0 -1.2566 -1.2566 0 0]
      | sbobj.Groups.Signals(12).Name = 'Signal 12'
      | sbobj.Groups.Signals(12).XData = [0 565 565.2 569.8 570 605]
      | sbobj.Groups.Signals(12).YData = [0 0 1.2566 1.2566 0 0]
      | sbobj.Groups.Signals(13).Name = 'Signal 13'
      | sbobj.Groups.Signals(13).XData = [0 575 575.2 579.8 580 605]
      | sbobj.Groups.Signals(13).YData = [0 0 -1.2566 -1.2566 0 0]
      | sbobj.Groups.Signals(14).Name = 'Signal 14'
      | sbobj.Groups.Signals(14).XData = [0 585 585.2 589.8 590 605]
      | sbobj.Groups.Signals(14).YData = [0 0 1.2566 1.2566 0 0]
      | sbobj.Groups.Signals(15).Name = 'Signal 15'
      | sbobj.Groups.Signals(15).XData = [0 595 595.2 599.8 600 605]
      | sbobj.Groups.Signals(15).YData = [0 0 -1.2566 -1.2566 0 0]
      | sbobj.Groups.TimeRange = [0 605]
  Signal 1 : Outport  Tag=STV Outport
  Signal 2 : Outport  Tag=STV Outport  Port=2
  Signal 3 : Outport  Tag=STV Outport  Port=3
  Signal 4 : Outport  Tag=STV Outport  Port=4
  Signal 5 : Outport  Tag=STV Outport  Port=5
  Signal 6 : Outport  Tag=STV Outport  Port=6
  Signal 7 : Outport  Tag=STV Outport  Port=7
  Signal 8 : Outport  Tag=STV Outport  Port=8
  Signal 9 : Outport  Tag=STV Outport  Port=9
  Signal 10 : Outport  Tag=STV Outport  Port=10
  Signal 11 : Outport  Tag=STV Outport  Port=11
  Signal 12 : Outport  Tag=STV Outport  Port=12
  Signal 13 : Outport  Tag=STV Outport  Port=13
  Signal 14 : Outport  Tag=STV Outport  Port=14
  Signal 15 : Outport  Tag=STV Outport  Port=15
  wires:
  FromWs/1 -> Demux/1
  Demux/1 -> Signal 1/1
  Demux/2 -> Signal 2/1
  Demux/3 -> Signal 3/1
  Demux/4 -> Signal 4/1
  Demux/5 -> Signal 5/1
  Demux/6 -> Signal 6/1
  Demux/7 -> Signal 7/1
  Demux/8 -> Signal 8/1
  Demux/9 -> Signal 9/1
  Demux/10 -> Signal 10/1
  Demux/11 -> Signal 11/1
  Demux/12 -> Signal 12/1
  Demux/13 -> Signal 13/1
  Demux/14 -> Signal 14/1
  Demux/15 -> Signal 15/1

== matlab function diagrama_completo/Completo con w finito/Subsistema Fisico/T.Park Dir ==
  data: fa input; fq output; fb input; fc input; theta_m input; fd output; f0 output
function [fq,fd,f0] = fcn(fa,fb,fc,theta_m)
fq=2/3*(cos(theta_m)*fa+cos(theta_m-(2*pi/(3)))*fb+cos(theta_m+(2*pi/(3)))*fc);
fd=2/3*(sin(theta_m)*fa+sin(theta_m-(2*pi/(3)))*fb+sin(theta_m+(2*pi/(3)))*fc);
f0=2/3*((1/2)*fa+(1/2)*fb+(1/2)*fc);

== matlab function diagrama_completo/Completo con w finito/Subsistema Fisico/T.Park Inv ==
  data: fq input; fa output; fd input; f0 input; theta_m input; fb output; fc output
function [fa,fb,fc] = fcn(fq,fd,f0,theta_m)
fa=fq*cos(theta_m)+fd*sin(theta_m)+f0;
fb=fq*cos(theta_m-(2*pi/(3)))+fd*sin(theta_m-(2*pi/(3)))+f0;
fc=fq*cos(theta_m+(2*pi/(3)))+fd*sin(theta_m+(2*pi/(3)))+f0;

== matlab function diagrama_completo/Completo con w finito/T.Park Dir ==
  data: fa input; fq output; fb input; fc input; theta_m input; fd output; f0 output
function [fq,fd,f0] = fcn(fa,fb,fc,theta_m)
fq=2/3*(cos(theta_m)*fa+cos(theta_m-(2*pi/(3)))*fb+cos(theta_m+(2*pi/(3)))*fc);
fd=2/3*(sin(theta_m)*fa+sin(theta_m-(2*pi/(3)))*fb+sin(theta_m+(2*pi/(3)))*fc);
f0=2/3*((1/2)*fa+(1/2)*fb+(1/2)*fc);

== matlab function diagrama_completo/Completo con w finito/T.Park Inv ==
  data: fq input; fa output; fd input; f0 input; theta_m input; fb output; fc output
function [fa,fb,fc] = fcn(fq,fd,f0,theta_m)
fa=fq*cos(theta_m)+fd*sin(theta_m)+f0;
fb=fq*cos(theta_m-(2*pi/(3)))+fd*sin(theta_m-(2*pi/(3)))+f0;
fc=fq*cos(theta_m+(2*pi/(3)))+fd*sin(theta_m+(2*pi/(3)))+f0;

== matlab function diagrama_completo/Completo con w infinito/Subsistema Fisico/T.Park Dir ==
  data: fa input; fq output; fb input; fc input; theta_m input; fd output; f0 output
function [fq,fd,f0] = fcn(fa,fb,fc,theta_m)
fq=2/3*(cos(theta_m)*fa+cos(theta_m-(2*pi/(3)))*fb+cos(theta_m+(2*pi/(3)))*fc);
fd=2/3*(sin(theta_m)*fa+sin(theta_m-(2*pi/(3)))*fb+sin(theta_m+(2*pi/(3)))*fc);
f0=2/3*((1/2)*fa+(1/2)*fb+(1/2)*fc);

== matlab function diagrama_completo/Completo con w infinito/Subsistema Fisico/T.Park Inv ==
  data: fq input; fa output; fd input; f0 input; theta_m input; fb output; fc output
function [fa,fb,fc] = fcn(fq,fd,f0,theta_m)
fa=fq*cos(theta_m)+fd*sin(theta_m)+f0;
fb=fq*cos(theta_m-(2*pi/(3)))+fd*sin(theta_m-(2*pi/(3)))+f0;
fc=fq*cos(theta_m+(2*pi/(3)))+fd*sin(theta_m+(2*pi/(3)))+f0;

== matlab function diagrama_completo/Completo con w infinito/T.Park Dir ==
  data: fa input; fq output; fb input; fc input; theta_m input; fd output; f0 output
function [fq,fd,f0] = fcn(fa,fb,fc,theta_m)
fq=2/3*(cos(theta_m)*fa+cos(theta_m-(2*pi/(3)))*fb+cos(theta_m+(2*pi/(3)))*fc);
fd=2/3*(sin(theta_m)*fa+sin(theta_m-(2*pi/(3)))*fb+sin(theta_m+(2*pi/(3)))*fc);
f0=2/3*((1/2)*fa+(1/2)*fb+(1/2)*fc);

== matlab function diagrama_completo/Completo con w infinito/T.Park Inv ==
  data: fq input; fa output; fd input; f0 input; theta_m input; fb output; fc output
function [fa,fb,fc] = fcn(fq,fd,f0,theta_m)
fa=fq*cos(theta_m)+fd*sin(theta_m)+f0;
fb=fq*cos(theta_m-(2*pi/(3)))+fd*sin(theta_m-(2*pi/(3)))+f0;
fc=fq*cos(theta_m+(2*pi/(3)))+fd*sin(theta_m+(2*pi/(3)))+f0;
